simulink model "all_together_simu_v1"  (R2020b)
settings: Solver=FixedStepDiscrete  StartTime=0.0  StopTime=simTime  RelTol=1e-3
InitFcn:
  | generate_locals_for_simulink
values from neighbouring files (symbols this model uses):
  Hh = abs(V(:,1)'*sqrt(S(1,1)))    [setup_old.m]
  Hv = abs(U(:,1)*sqrt(S(1,1)))    [setup_old.m]
undefined symbols (not defined in the file or in its folder): gray, magnitude, Rec, SDTV
libraries: hdlsllib x52, simulink x15, visionhdlio x11, visionsinks x7, visionhdlutilities x4, visionconversions x1, visionsources x1
(part 1 of 2)
settings Model: DataTypeOverride=Off  SimulationMode=accelerator  Creator=The MathWorks, Inc.  LastModifiedBy=Ethan
settings SolverCC: AutoInsertRateTranBlk=on
settings DataIOCC: LimitDataPoints=on  SaveOutput=off  SignalLogging=off  SaveTime=off  ReturnWorkspaceOutputs=off
settings OptimizationCC: BlockReduction=off  ConditionallyExecuteInputs=off  DefaultParameterBehavior=Inlined  LifeSpan=inf
settings DebuggingCC: AlgebraicLoopMsg=error  SingleTaskRateTransMsg=error  ParameterPrecisionLossMsg=none  AllowSymbolicDim=off  StrictBusMsg=ErrorOnBusTreatedAsVector  SFUnexpectedBacktrackingDiag=warning  SFNoUnconditionalDefaultTransitionDiag=warning  SFExecutionAtInitializationDiag=none  ArithmeticOperatorsInVariantConditions=warning
settings HardwareCC: ProdBitPerPointer=32  ProdBitPerSizeT=32  ProdBitPerPtrDiffT=32  ProdLargestAtomicFloat=None  ProdIntDivRoundTo=Undefined  ProdEndianess=Unspecified  ProdWordSize=32  ProdHWDeviceType=ASIC/FPGA->ASIC/FPGA  ProdEqTarget=off
settings SFSimCC: SimUseLocalCustomCode=off  CustomCodeUndefinedFunction=UseInterfaceOnly
settings RTWCC: RTWUseLocalCustomCode=off
settings CodeAppCC: StateflowObjectComments=on
settings GRTTargetCC: TargetLangStandard=C89/C90 (ANSI)
settings ConfigComp: CovMetricSettings=dw  CovSaveCumulativeToWorkspaceVar=on  CovSaveSingleToWorkspaceVar=on  CovExternalEMLEnable=off  CovSFcnEnable=off

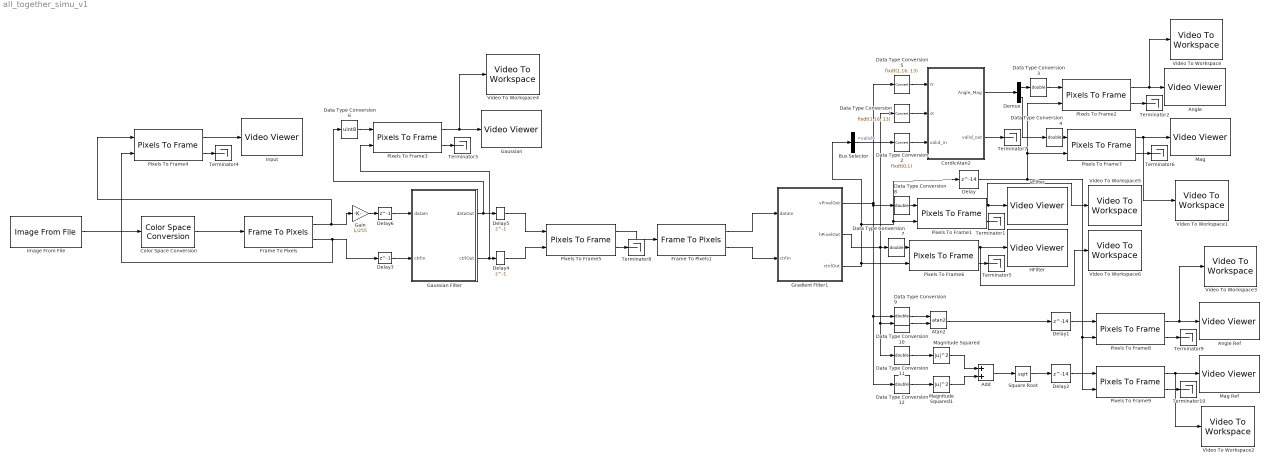
== system all_together_simu_v1 ==
  Add : Sum
  Angle : VideoViewer  colormapValue=gray(256)  FigPos=[1922 517 909 409]
  Angle Ref : VideoViewer  FigPos=[2808 517 958 409]
  Atan2 : Trigonometry  Operator=atan2  ApproximationMethod=CORDIC  NumberOfIterations=12
  Bus Selector : BusSelector  OutputSignals=valid
  Color Space Conversion : visionconversions/Color Space  Conversion  conversion=Obsolete  conversionActive=R'G'B' to intensity  wp_str=D65  rec=Rec. 601 (SDTV)  sys=1125/60/2:1  imagePorts=One multidimensional signal
  CordicAtan2 : Subsystem
  Data Type Conversion1 : DataTypeConversion  OutMin=0  OutMax=1  OutDataTypeStr=fixdt(1,16, 13)
  Data Type Conversion{7..12} (6 alike) : DataTypeConversion  OutMin=0  OutMax=1  OutDataTypeStr=double
  Data Type Conversion2 : DataTypeConversion  OutMin=0  OutMax=1  OutDataTypeStr=fixdt(0,1)
  Data Type Conversion3 : DataTypeConversion  OutDataTypeStr=double
  Data Type Conversion4 : DataTypeConversion  OutDataTypeStr=double
  Data Type Conversion5 : DataTypeConversion  OutMin=0  OutMax=1  OutDataTypeStr=fixdt(1,16, 13)
  Data Type Conversion6 : DataTypeConversion  OutMin=0  OutMax=1  OutDataTypeStr=uint8
  Delay : Delay  DelayLength=14
  Delay1 : Delay  DelayLength=14
  Delay2 : Delay  DelayLength=14
  Delay{3..6} (4 alike) : Delay  DelayLength=1
  Demux : Demux  Outputs=2
  Frame To Pixels : visionhdlio/Frame To Pixels  NumComponents=1  NumPixels=1  VideoFormat=480p  ActivePixelsPerLine=32  ActiveVideoLines=18  TotalPixelsPerLine=42  TotalVideoLines=28  StartingActiveLine=6  FrontPorch=5  SampleTime=0
      settings: SourceProductName=Vision HDL Toolbox
  Frame To Pixels1 : visionhdlio/Frame To Pixels  NumComponents=1  NumPixels=1  VideoFormat=480p  ActivePixelsPerLine=32  ActiveVideoLines=18  TotalPixelsPerLine=42  TotalVideoLines=28  StartingActiveLine=6  FrontPorch=5  SampleTime=0
      settings: SourceProductName=Vision HDL Toolbox
  Gain : Gain  Gain=1/255  OutDataTypeStr=fixdt(1,16, 14)
  Gaussian : VideoViewer  FigPos=[2900 799 813 623.666666666667]
  Gaussian Filter : Subsystem
  Gradient Filter1 : Subsystem
  HFilter : VideoViewer  FigPos=[2895 936 813 624]
  Image From File : visionsources/Image From File  Tag=vipblks_nd  FileName=start.png  Ts=1  imagePorts=One multidimensional signal  OutPortLabels=R|G|B  ImageDataType=uint8  sdImageDataType=uint(8)  Signed=on  WordLength=16  FractionLengthMode=User-defined  FractionLength=15
  Input : VideoViewer  FigPos=[170 848 670 624]
  Mag : VideoViewer  FigPos=[1914 1017 954 411]
  Mag Ref : VideoViewer  FigPos=[2855 1015 954 411]
  Magnitude Squared : Math  Operator=magnitude^2  SaturateOnIntegerOverflow=on
  Magnitude Squared1 : Math  Operator=magnitude^2  SaturateOnIntegerOverflow=on
  Pixels To Frame{1..9} (9 alike) : visionhdlio/Pixels To Frame  NumComponents=1  NumPixels=1  VideoFormat=480p  ActivePixelsPerLine=32  ActiveVideoLines=18  TotalPixelsPerLine=42  TotalVideoLines=28
      settings: SourceProductBaseCode=VT
  Square Root : Sqrt  SaturateOnIntegerOverflow=on
  Terminator{1..10} (10 alike) : Terminator
  VFilter : VideoViewer  FigPos=[928 938 813 624]
  Video To Workspace : visionsinks/Video To Workspace  VariableName=angle  NumInputs=1  DataLimit=10  DecimationFactor=1  LogFi=off  InPortLabels=R|G|B
      settings: SourceProductBaseCode=VP
  Video To Workspace1 : visionsinks/Video To Workspace  VariableName=mag  NumInputs=1  DataLimit=10  DecimationFactor=1  LogFi=off  InPortLabels=R|G|B
      settings: SourceProductBaseCode=VP
  Video To Workspace2 : visionsinks/Video To Workspace  VariableName=mag_ref  NumInputs=1  DataLimit=10  DecimationFactor=1  LogFi=off  InPortLabels=R|G|B
      settings: SourceProductBaseCode=VP
  Video To Workspace3 : visionsinks/Video To Workspace  VariableName=angle_ref  NumInputs=1  DataLimit=10  DecimationFactor=1  LogFi=off  InPortLabels=R|G|B
      settings: SourceProductBaseCode=VP
  Video To Workspace4 : visionsinks/Video To Workspace  VariableName=gaussian  NumInputs=1  DataLimit=10  DecimationFactor=1  LogFi=off  InPortLabels=R|G|B
      settings: SourceProductBaseCode=VP
  Video To Workspace5 : visionsinks/Video To Workspace  VariableName=iy  NumInputs=1  DataLimit=10  DecimationFactor=1  LogFi=off  InPortLabels=R|G|B
      settings: SourceProductBaseCode=VP
  Video To Workspace6 : visionsinks/Video To Workspace  VariableName=ix  NumInputs=1  DataLimit=10  DecimationFactor=1  LogFi=off  InPortLabels=R|G|B
      settings: SourceProductBaseCode=VP
  wires:
  Delay6/1 -> Gaussian Filter/1(dataIn)
  Delay3/1 -> Gaussian Filter/2(ctrlIn)
  Gaussian Filter/2(ctrlOut) -> Pixels To Frame3/2, Delay4/1
  Frame To Pixels/2 -> Pixels To Frame4/2, Delay3/1
  Pixels To Frame3/1 -> Video To Workspace4/1, Gaussian/1
  Pixels To Frame3/2 -> Terminator3/1
  Gaussian Filter/1(dataOut) -> Data Type Conversion6/1, Delay5/1
  Pixels To Frame4/2 -> Terminator4/1
  Pixels To Frame4/1 -> Input/1
  Frame To Pixels/1 -> Pixels To Frame4/1, Gain/1
  Pixels To Frame1/2 -> Terminator1/1
  Pixels To Frame1/1 -> Video To Workspace5/1, VFilter/1
  Gradient Filter1/3(ctrilOut) -> Pixels To Frame6/2, Bus Selector/1, Delay/1, Pixels To Frame1/2
  Delay5/1 -> Pixels To Frame5/1
  Delay4/1 -> Pixels To Frame5/2
  Pixels To Frame5/1 -> Frame To Pixels1/1
  Frame To Pixels1/1 -> Gradient Filter1/1(dataIn)
  Frame To Pixels1/2 -> Gradient Filter1/2(ctrlIn)
  Pixels To Frame6/1 -> HFilter/1, Video To Workspace6/1
  Pixels To Frame6/2 -> Terminator5/1
  Bus Selector/1 -> Data Type Conversion2/1  "<valid>"
  Pixels To Frame2/2 -> Terminator2/1
  Pixels To Frame2/1 -> Video To Workspace/1, Angle/1
  CordicAtan2/1(Angle_Mag) -> Demux/1
  Demux/1 -> Data Type Conversion3/1
  Pixels To Frame7/2 -> Terminator6/1
  Pixels To Frame7/1 -> Video To Workspace1/1, Mag/1
  Demux/2 -> Data Type Conversion4/1
  Delay/1 -> Pixels To Frame9/2, Pixels To Frame8/2, Pixels To Frame2/2, Pixels To Frame7/2
  CordicAtan2/2(valid_out) -> Terminator7/1
  Pixels To Frame5/2 -> Terminator8/1
  Data Type Conversion3/1 -> Pixels To Frame2/1
  Data Type Conversion4/1 -> Pixels To Frame7/1
  Gain/1 -> Delay6/1
  Data Type Conversion2/1 -> CordicAtan2/3(valid_in)
  Atan2/1 -> Delay1/1
  Magnitude Squared/1 -> Add/1
  Magnitude Squared1/1 -> Add/2
  Add/1 -> Square Root/1
  Square Root/1 -> Delay2/1
  Delay2/1 -> Pixels To Frame9/1
  Delay1/1 -> Pixels To Frame8/1
  Pixels To Frame9/1 -> Video To Workspace2/1, Mag Ref/1
  Pixels To Frame8/1 -> Video To Workspace3/1, Angle Ref/1
  Pixels To Frame8/2 -> Terminator9/1
  Pixels To Frame9/2 -> Terminator10/1
  Image From File/1 -> Color Space Conversion/1
  Color Space Conversion/1 -> Frame To Pixels/1
  Gradient Filter1/2(hPixelOut) -> Data Type Conversion1/1, Data Type Conversion7/1, Data Type Conversion11/1, Data Type Conversion10/1
  Gradient Filter1/1(vPixelOut) -> Data Type Conversion5/1, Data Type Conversion8/1, Data Type Conversion9/1, Data Type Conversion12/1
  Data Type Conversion6/1 -> Pixels To Frame3/1
  Data Type Conversion7/1 -> Pixels To Frame6/1
  Data Type Conversion8/1 -> Pixels To Frame1/1
  Data Type Conversion9/1 -> Atan2/1
  Data Type Conversion10/1 -> Atan2/2
  Data Type Conversion11/1 -> Magnitude Squared/1
  Data Type Conversion12/1 -> Magnitude Squared1/1
  Data Type Conversion1/1 -> CordicAtan2/2(iX)
  Data Type Conversion5/1 -> CordicAtan2/1(iY)

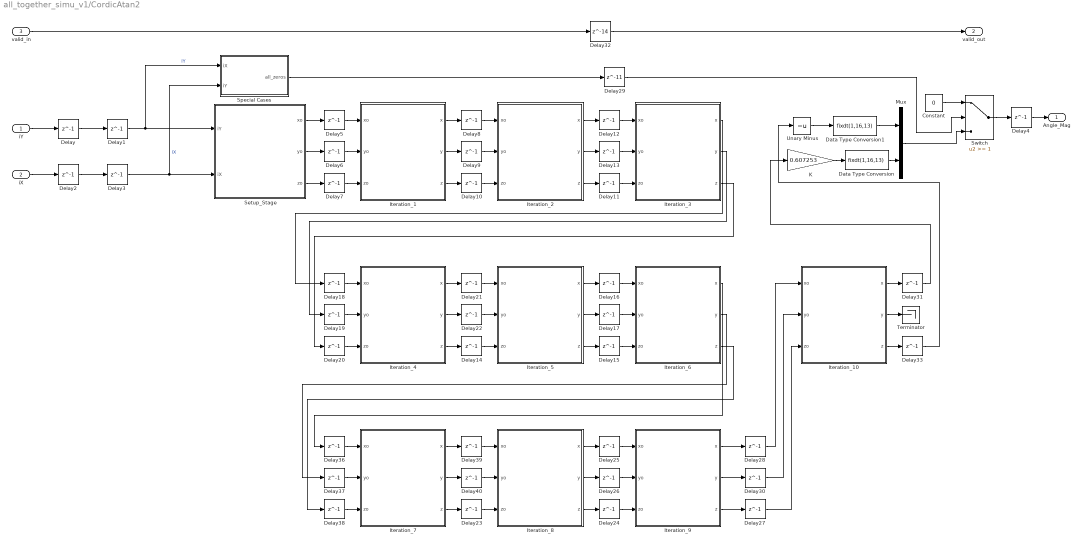
== system all_together_simu_v1/CordicAtan2 ==
  iY : Inport
  iX : Inport  Port=2
  valid_in : Inport  Port=3  OutMin=[0]  OutMax=[1]  OutDataTypeStr=fixdt(0,1)
  Constant : Constant  Value=0  OutDataTypeStr=fixdt(1,16,14)  SampleTime=-1
  Data Type Conversion : DataTypeConversion  OutDataTypeStr=fixdt(1,16,13)
  Data Type Conversion1 : DataTypeConversion  OutDataTypeStr=fixdt(1,16,13)
  Delay{,1..28,30..31,33,36..40} (37 alike) : Delay  DelayLength=1
  Delay29 : Delay  DelayLength=11
  Delay32 : Delay  DelayLength=14
  Iteration_1 : Subsystem
  Iteration_10 : Subsystem
  Iteration_2 : Subsystem
  Iteration_3 : Subsystem
  Iteration_4 : Subsystem
  Iteration_5 : Subsystem
  Iteration_6 : Subsystem
  Iteration_7 : Subsystem
  Iteration_8 : Subsystem
  Iteration_9 : Subsystem
  K : Gain  Gain=0.607253  OutDataTypeStr=Inherit: Inherit via back propagation
  Mux : Mux  Inputs=2
  Setup_Stage : Subsystem
  Special Cases : Subsystem
  Switch : Switch  Threshold=1
  Terminator : Terminator
  Unary Minus : UnaryMinus
  Angle_Mag : Outport
  valid_out : Outport  Port=2  OutMin=[0]  OutMax=[1]  OutDataTypeStr=fixdt(0,1)
  wires:
  iY/1 -> Delay/1
  Delay/1 -> Delay1/1
  Delay2/1 -> Delay3/1
  iX/1 -> Delay2/1
  Constant/1 -> Switch/1
  Delay4/1 -> Angle_Mag/1
  Switch/1 -> Delay4/1
  Delay1/1 -> Setup_Stage/1(iY), Special Cases/1(iX)  "iY"
  Delay3/1 -> Special Cases/2(iY), Setup_Stage/2(iX)  "iX"
  Special Cases/1(all_zeros) -> Delay29/1
  Setup_Stage/1(xo) -> Delay5/1
  Setup_Stage/2(yo) -> Delay6/1
  Setup_Stage/3(zo) -> Delay7/1
  Delay7/1 -> Iteration_1/3(zo)
  Delay6/1 -> Iteration_1/2(yo)
  Delay5/1 -> Iteration_1/1(xo)
  Iteration_1/3(z) -> Delay10/1
  Iteration_1/1(x) -> Delay8/1
  Iteration_1/2(y) -> Delay9/1
  Delay9/1 -> Iteration_2/2(yo)
  Delay10/1 -> Iteration_2/3(zo)
  Delay8/1 -> Iteration_2/1(xo)
  Delay11/1 -> Iteration_3/3(zo)
  Delay12/1 -> Iteration_3/1(xo)
  Delay13/1 -> Iteration_3/2(yo)
  Iteration_2/2(y) -> Delay13/1
  Iteration_2/1(x) -> Delay12/1
  Iteration_2/3(z) -> Delay11/1
  Iteration_5/1(x) -> Delay16/1
  Iteration_5/2(y) -> Delay17/1
  Delay16/1 -> Iteration_6/1(xo)
  Delay17/1 -> Iteration_6/2(yo)
  Delay15/1 -> Iteration_6/3(zo)
  Iteration_5/3(z) -> Delay15/1
  Iteration_4/3(z) -> Delay14/1
  Delay14/1 -> Iteration_5/3(zo)
  Iteration_4/2(y) -> Delay22/1
  Delay21/1 -> Iteration_5/1(xo)
  Delay18/1 -> Iteration_4/1(xo)
  Delay20/1 -> Iteration_4/3(zo)
  Iteration_4/1(x) -> Delay21/1
  Delay22/1 -> Iteration_5/2(yo)
  Delay19/1 -> Iteration_4/2(yo)
  Iteration_8/1(x) -> Delay25/1
  Iteration_8/2(y) -> Delay26/1
  Delay25/1 -> Iteration_9/1(xo)
  Delay26/1 -> Iteration_9/2(yo)
  Delay24/1 -> Iteration_9/3(zo)
  Iteration_8/3(z) -> Delay24/1
  Iteration_7/3(z) -> Delay23/1
  Delay23/1 -> Iteration_8/3(zo)
  Iteration_7/2(y) -> Delay40/1
  Delay39/1 -> Iteration_8/1(xo)
  Delay36/1 -> Iteration_7/1(xo)
  Delay38/1 -> Iteration_7/3(zo)
  Iteration_7/1(x) -> Delay39/1
  Delay40/1 -> Iteration_8/2(yo)
  Delay37/1 -> Iteration_7/2(yo)
  Iteration_3/3(z) -> Delay20/1
  Iteration_3/2(y) -> Delay19/1
  Iteration_3/1(x) -> Delay18/1
  Iteration_6/3(z) -> Delay38/1
  Iteration_6/2(y) -> Delay37/1
  Iteration_6/1(x) -> Delay36/1
  Iteration_9/2(y) -> Delay30/1
  Iteration_9/1(x) -> Delay28/1
  Iteration_9/3(z) -> Delay27/1
  Mux/1 -> Switch/3
  Delay29/1 -> Switch/2
  Delay28/1 -> Iteration_10/1(xo)
  Delay30/1 -> Iteration_10/2(yo)
  Delay27/1 -> Iteration_10/3(zo)
  Iteration_10/1(x) -> Delay31/1
  Delay31/1 -> K/1
  Iteration_10/2(y) -> Terminator/1
  Iteration_10/3(z) -> Delay33/1
  Delay33/1 -> Unary Minus/1
  Unary Minus/1 -> Data Type Conversion1/1
  valid_in/1 -> Delay32/1
  Delay32/1 -> valid_out/1
  Data Type Conversion/1 -> Mux/2
  K/1 -> Data Type Conversion/1
  Data Type Conversion1/1 -> Mux/1

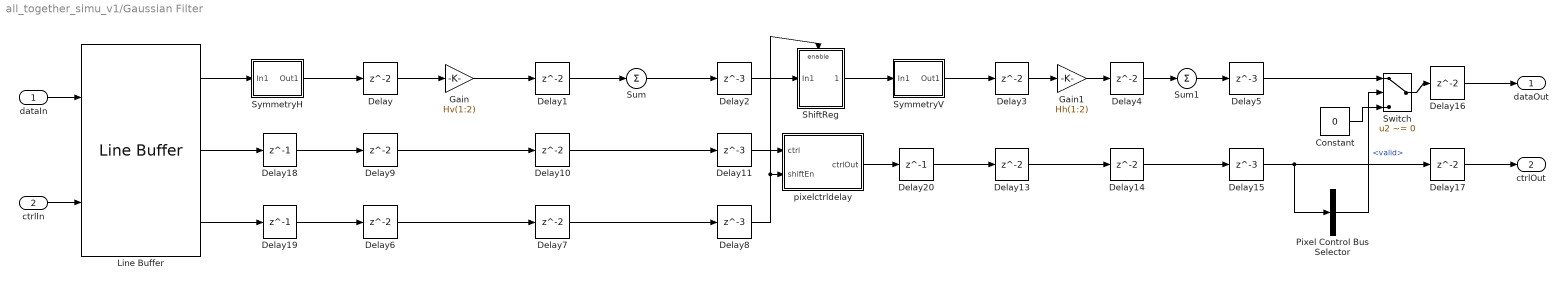
== system all_together_simu_v1/Gaussian Filter ==
  dataIn : Inport
  ctrlIn : Inport  Port=2
  Constant : Constant  Value=0  OutDataTypeStr=Inherit: Inherit via back propagation  SampleTime=-1
  Delay{,1,3..4,6..7,9..10,13..14,16..17} (12 alike) : Delay
  Delay{2,5,8,11,15} (5 alike) : Delay  DelayLength=3
  Delay18 : Delay  DelayLength=1
  Delay19 : Delay  DelayLength=1
  Delay20 : Delay  DelayLength=1
  Gain : Gain  Gain=Hv(1:2)  ParamDataTypeStr=good_fixdt
  Gain1 : Gain  Gain=Hh(1:2)  ParamDataTypeStr=good_fixdt
  Line Buffer : visionhdlutilities/Line Buffer  NeighborhoodSize=[3 3]  PaddingMethod=None  PaddingValue=0  LineBufferSize=2048  SimulateUsing=Code generation
      settings: SourceProductName=Vision HDL Toolbox
  Pixel Control Bus Selector : BusSelector  OutputSignals=valid
  ShiftReg : Subsystem
  Sum : Sum  Inputs=1  OutDataTypeStr=Inherit: Same as accumulator
  Sum1 : Sum  Inputs=1  OutDataTypeStr=Inherit: Same as accumulator
  Switch : Switch  Criteria=u2 ~= 0
  SymmetryH : Subsystem
  SymmetryV : Subsystem
  pixelctrldelay : Subsystem
  dataOut : Outport  VectorParamsAs1DForOutWhenUnconnected=off
  ctrlOut : Outport  Port=2  VectorParamsAs1DForOutWhenUnconnected=off
  wires:
  Gain/1 -> Delay1/1
  Delay8/1 -> pixelctrldelay/2(shiftEn), ShiftReg/Enable
  Delay3/1 -> Gain1/1
  Sum/1 -> Delay2/1
  Gain1/1 -> Delay4/1
  Sum1/1 -> Delay5/1
  Delay9/1 -> Delay10/1
  dataIn/1 -> Line Buffer/1
  Delay10/1 -> Delay11/1
  Delay4/1 -> Sum1/1
  Delay6/1 -> Delay7/1
  Delay1/1 -> Sum/1
  Delay17/1 -> ctrlOut/1
  Constant/1 -> Switch/3
  Delay14/1 -> Delay15/1
  Delay13/1 -> Delay14/1
  Delay2/1 -> ShiftReg/1(In1)
  Delay7/1 -> Delay8/1
  Switch/1 -> Delay16/1
  Delay15/1 -> Delay17/1, Pixel Control Bus Selector/1
  Pixel Control Bus Selector/1 -> Switch/2  "<valid>"
  Delay/1 -> Gain/1
  ctrlIn/1 -> Line Buffer/2
  Delay16/1 -> dataOut/1
  Line Buffer/3 -> Delay19/1
  Line Buffer/2 -> Delay18/1
  ShiftReg/1(Out1) -> SymmetryV/1(In1)
  Line Buffer/1 -> SymmetryH/1(In1)
  SymmetryH/1(Out1) -> Delay/1
  Delay18/1 -> Delay9/1
  Delay19/1 -> Delay6/1
  SymmetryV/1(Out1) -> Delay3/1
  Delay20/1 -> Delay13/1
  Delay11/1 -> pixelctrldelay/1(ctrl)
  pixelctrldelay/1(ctrlOut) -> Delay20/1
  Delay5/1 -> Switch/1

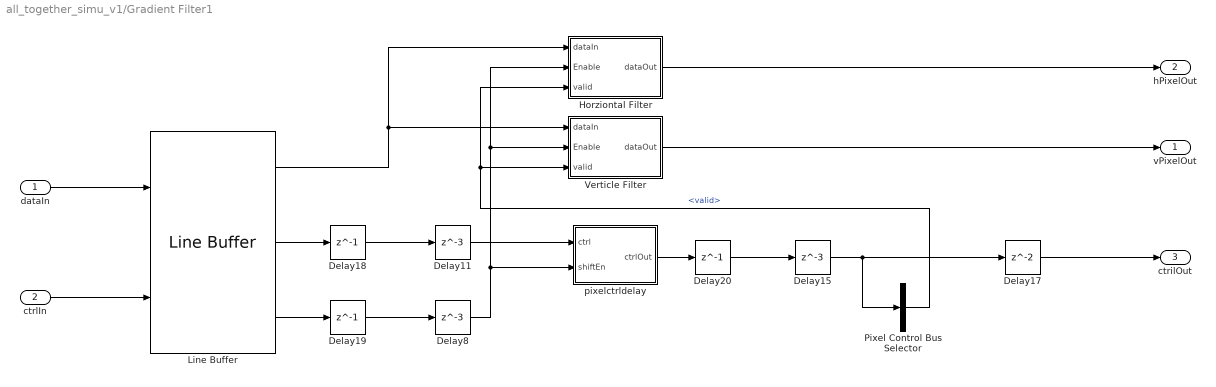
== system all_together_simu_v1/Gradient Filter1 ==
  dataIn : Inport
  ctrlIn : Inport  Port=2
  Delay11 : Delay  DelayLength=3
  Delay15 : Delay  DelayLength=3
  Delay17 : Delay
  Delay18 : Delay  DelayLength=1
  Delay19 : Delay  DelayLength=1
  Delay20 : Delay  DelayLength=1
  Delay8 : Delay  DelayLength=3
  Horziontal Filter : Subsystem
  Line Buffer : visionhdlutilities/Line Buffer  NeighborhoodSize=[3 3]  PaddingMethod=None  PaddingValue=0  LineBufferSize=2048  SimulateUsing=Code generation
      settings: SourceProductName=Vision HDL Toolbox
  Pixel Control Bus Selector : BusSelector  OutputSignals=valid
  Verticle Filter : Subsystem
  pixelctrldelay : Subsystem
  vPixelOut : Outport  VectorParamsAs1DForOutWhenUnconnected=off
  hPixelOut : Outport  Port=2  VectorParamsAs1DForOutWhenUnconnected=off
  ctrilOut : Outport  Port=3  VectorParamsAs1DForOutWhenUnconnected=off
  wires:
  ctrlIn/1 -> Line Buffer/2
  dataIn/1 -> Line Buffer/1
  Line Buffer/1 -> Horziontal Filter/1(dataIn), Verticle Filter/1(dataIn)
  Delay20/1 -> Delay15/1
  Delay19/1 -> Delay8/1
  Delay11/1 -> pixelctrldelay/1(ctrl)
  pixelctrldelay/1(ctrlOut) -> Delay20/1
  Delay15/1 -> Delay17/1, Pixel Control Bus Selector/1
  Delay18/1 -> Delay11/1
  Delay8/1 -> Horziontal Filter/2(Enable), Verticle Filter/2(Enable), pixelctrldelay/2(shiftEn)
  Line Buffer/2 -> Delay18/1
  Line Buffer/3 -> Delay19/1
  Pixel Control Bus Selector/1 -> Horziontal Filter/3(valid), Verticle Filter/3(valid)  "<valid>"
  Verticle Filter/1(dataOut) -> vPixelOut/1
  Horziontal Filter/1(dataOut) -> hPixelOut/1
  Delay17/1 -> ctrilOut/1

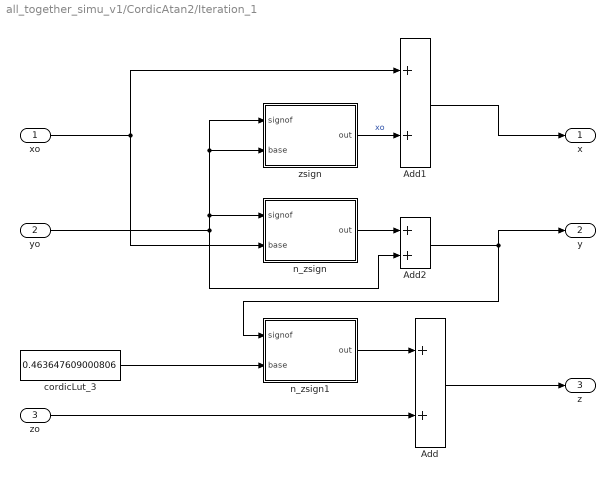
== system all_together_simu_v1/CordicAtan2/Iteration_1 ==
  xo : Inport
  yo : Inport  Port=2
  zo : Inport  Port=3
  Add : Sum
  Add1 : Sum
  Add2 : Sum
  cordicLut_3 : Constant  Value=0.463647609000806  OutDataTypeStr=fixdt(1,16,16)  SampleTime=-1
  n_zsign : Subsystem
  n_zsign1 : Subsystem
  zsign : Subsystem
  x : Outport
  y : Outport  Port=2
  z : Outport  Port=3
  wires:
  Add/1 -> z/1
  cordicLut_3/1 -> n_zsign1/2(base)
  zo/1 -> Add/2
  n_zsign1/1(out) -> Add/1
  yo/1 -> zsign/2(base), zsign/1(signof), n_zsign/1(signof), Add2/2
  zsign/1(out) -> Add1/2  "xo"
  xo/1 -> n_zsign/2(base), Add1/1
  Add1/1 -> x/1
  n_zsign/1(out) -> Add2/1
  Add2/1 -> n_zsign1/1(signof), y/1

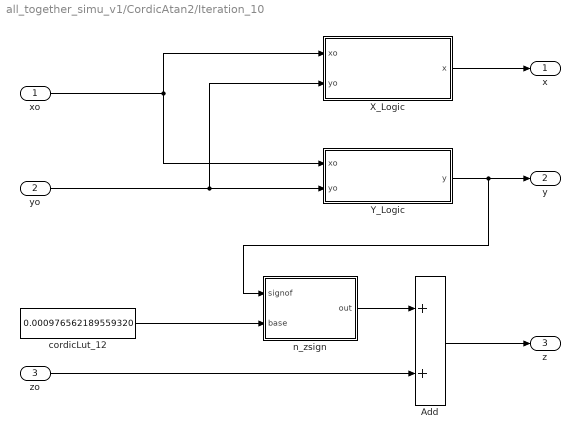
== system all_together_simu_v1/CordicAtan2/Iteration_10 ==
  xo : Inport
  yo : Inport  Port=2
  zo : Inport  Port=3
  Add : Sum
  X_Logic : Subsystem
  Y_Logic : Subsystem
  cordicLut_12 : Constant  Value=0.000976562189559320  OutDataTypeStr=fixdt(1,16,24)  SampleTime=-1
  n_zsign : Subsystem
  x : Outport
  y : Outport  Port=2
  z : Outport  Port=3
  wires:
  Add/1 -> z/1
  cordicLut_12/1 -> n_zsign/2(base)
  zo/1 -> Add/2
  n_zsign/1(out) -> Add/1
  yo/1 -> Y_Logic/2(yo), X_Logic/2(yo)
  xo/1 -> Y_Logic/1(xo), X_Logic/1(xo)
  X_Logic/1(x) -> x/1
  Y_Logic/1(y) -> n_zsign/1(signof), y/1

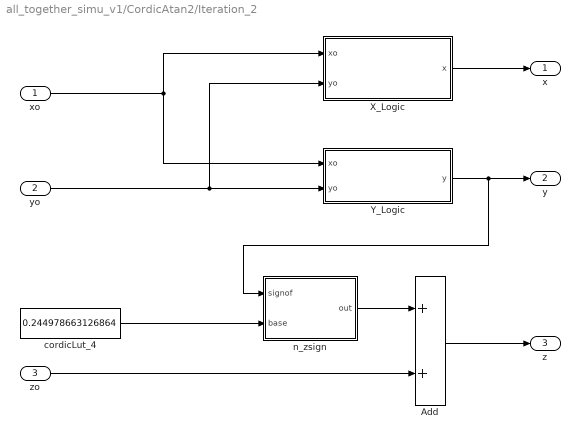
== system all_together_simu_v1/CordicAtan2/Iteration_2 ==
  xo : Inport
  yo : Inport  Port=2
  zo : Inport  Port=3
  Add : Sum
  X_Logic : Subsystem
  Y_Logic : Subsystem
  cordicLut_4 : Constant  Value=0.244978663126864  OutDataTypeStr=fixdt(1,16, 17)  SampleTime=-1
  n_zsign : Subsystem
  x : Outport
  y : Outport  Port=2
  z : Outport  Port=3
  wires:
  Add/1 -> z/1
  cordicLut_4/1 -> n_zsign/2(base)
  zo/1 -> Add/2
  n_zsign/1(out) -> Add/1
  yo/1 -> Y_Logic/2(yo), X_Logic/2(yo)
  xo/1 -> Y_Logic/1(xo), X_Logic/1(xo)
  X_Logic/1(x) -> x/1
  Y_Logic/1(y) -> n_zsign/1(signof), y/1

== system all_together_simu_v1/CordicAtan2/Iteration_3 ==
  xo : Inport
  yo : Inport  Port=2
  zo : Inport  Port=3
  Add : Sum
  X_Logic : Subsystem
  Y_Logic : Subsystem
  cordicLut_5 : Constant  Value=0.124354994546761  OutDataTypeStr=fixdt(1,16,17)  SampleTime=-1
  n_zsign : Subsystem
  x : Outport
  y : Outport  Port=2
  z : Outport  Port=3
  wires:
  Add/1 -> z/1
  cordicLut_5/1 -> n_zsign/2(base)
  zo/1 -> Add/2
  n_zsign/1(out) -> Add/1
  yo/1 -> Y_Logic/2(yo), X_Logic/2(yo)
  xo/1 -> Y_Logic/1(xo), X_Logic/1(xo)
  X_Logic/1(x) -> x/1
  Y_Logic/1(y) -> n_zsign/1(signof), y/1

== system all_together_simu_v1/CordicAtan2/Iteration_4 ==
  xo : Inport
  yo : Inport  Port=2
  zo : Inport  Port=3
  Add : Sum
  X_Logic : Subsystem
  Y_Logic : Subsystem
  cordicLut_6 : Constant  Value=0.0624188099959574  OutDataTypeStr=fixdt(1,16,18)  SampleTime=-1
  n_zsign : Subsystem
  x : Outport
  y : Outport  Port=2
  z : Outport  Port=3
  wires:
  Add/1 -> z/1
  cordicLut_6/1 -> n_zsign/2(base)
  zo/1 -> Add/2
  n_zsign/1(out) -> Add/1
  yo/1 -> Y_Logic/2(yo), X_Logic/2(yo)
  xo/1 -> Y_Logic/1(xo), X_Logic/1(xo)
  X_Logic/1(x) -> x/1
  Y_Logic/1(y) -> n_zsign/1(signof), y/1

== system all_together_simu_v1/CordicAtan2/Iteration_5 ==
  xo : Inport
  yo : Inport  Port=2
  zo : Inport  Port=3
  Add : Sum
  X_Logic : Subsystem
  Y_Logic : Subsystem
  cordicLut_7 : Constant  Value=0.0312398334302683  OutDataTypeStr=fixdt(1,16,19)  SampleTime=-1
  n_zsign : Subsystem
  x : Outport
  y : Outport  Port=2
  z : Outport  Port=3
  wires:
  Add/1 -> z/1
  cordicLut_7/1 -> n_zsign/2(base)
  zo/1 -> Add/2
  n_zsign/1(out) -> Add/1
  yo/1 -> Y_Logic/2(yo), X_Logic/2(yo)
  xo/1 -> Y_Logic/1(xo), X_Logic/1(xo)
  X_Logic/1(x) -> x/1
  Y_Logic/1(y) -> n_zsign/1(signof), y/1

== system all_together_simu_v1/CordicAtan2/Iteration_6 ==
  xo : Inport
  yo : Inport  Port=2
  zo : Inport  Port=3
  Add : Sum
  X_Logic : Subsystem
  Y_Logic : Subsystem
  cordicLut_8 : Constant  Value=0.0156237286204768  OutDataTypeStr=fixdt(1,16,20)  SampleTime=-1
  n_zsign : Subsystem
  x : Outport
  y : Outport  Port=2
  z : Outport  Port=3
  wires:
  Add/1 -> z/1
  cordicLut_8/1 -> n_zsign/2(base)
  zo/1 -> Add/2
  n_zsign/1(out) -> Add/1
  yo/1 -> Y_Logic/2(yo), X_Logic/2(yo)
  xo/1 -> Y_Logic/1(xo), X_Logic/1(xo)
  X_Logic/1(x) -> x/1
  Y_Logic/1(y) -> n_zsign/1(signof), y/1

== system all_together_simu_v1/CordicAtan2/Iteration_7 ==
  xo : Inport
  yo : Inport  Port=2
  zo : Inport  Port=3
  Add : Sum
  X_Logic : Subsystem
  Y_Logic : Subsystem
  cordicLut_9 : Constant  Value=0.00781234106010111  OutDataTypeStr=fixdt(1,16,21)  SampleTime=-1
  n_zsign : Subsystem
  x : Outport
  y : Outport  Port=2
  z : Outport  Port=3
  wires:
  Add/1 -> z/1
  cordicLut_9/1 -> n_zsign/2(base)
  zo/1 -> Add/2
  n_zsign/1(out) -> Add/1
  yo/1 -> Y_Logic/2(yo), X_Logic/2(yo)
  xo/1 -> Y_Logic/1(xo), X_Logic/1(xo)
  X_Logic/1(x) -> x/1
  Y_Logic/1(y) -> n_zsign/1(signof), y/1

== system all_together_simu_v1/CordicAtan2/Iteration_8 ==
  xo : Inport
  yo : Inport  Port=2
  zo : Inport  Port=3
  Add : Sum
  X_Logic : Subsystem
  Y_Logic : Subsystem
  cordicLut_10 : Constant  Value=0.00390623013196697  OutDataTypeStr=fixdt(1,16,22)  SampleTime=-1
  n_zsign : Subsystem
  x : Outport
  y : Outport  Port=2
  z : Outport  Port=3
  wires:
  Add/1 -> z/1
  cordicLut_10/1 -> n_zsign/2(base)
  zo/1 -> Add/2
  n_zsign/1(out) -> Add/1
  yo/1 -> Y_Logic/2(yo), X_Logic/2(yo)
  xo/1 -> Y_Logic/1(xo), X_Logic/1(xo)
  X_Logic/1(x) -> x/1
  Y_Logic/1(y) -> n_zsign/1(signof), y/1

== system all_together_simu_v1/CordicAtan2/Iteration_9 ==
  xo : Inport
  yo : Inport  Port=2
  zo : Inport  Port=3
  Add : Sum
  X_Logic : Subsystem
  Y_Logic : Subsystem
  cordicLut_11 : Constant  Value=0.00195312251647882  OutDataTypeStr=fixdt(1,16,23)  SampleTime=-1
  n_zsign : Subsystem
  x : Outport
  y : Outport  Port=2
  z : Outport  Port=3
  wires:
  Add/1 -> z/1
  cordicLut_11/1 -> n_zsign/2(base)
  zo/1 -> Add/2
  n_zsign/1(out) -> Add/1
  yo/1 -> Y_Logic/2(yo), X_Logic/2(yo)
  xo/1 -> Y_Logic/1(xo), X_Logic/1(xo)
  X_Logic/1(x) -> x/1
  Y_Logic/1(y) -> n_zsign/1(signof), y/1

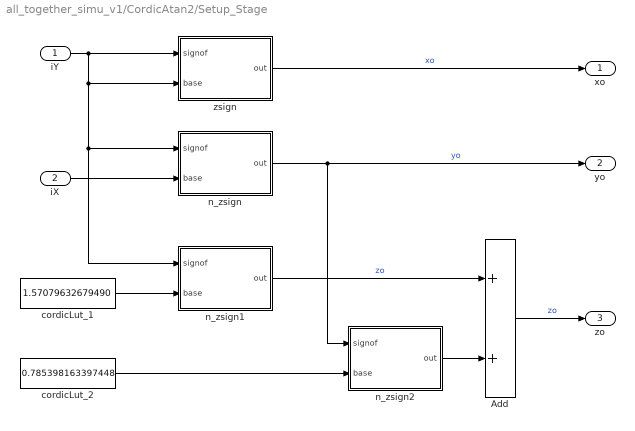
== system all_together_simu_v1/CordicAtan2/Setup_Stage ==
  iY : Inport
  iX : Inport  Port=2
  Add : Sum
  cordicLut_1 : Constant  Value=1.57079632679490  OutDataTypeStr=fixdt(1,16, 14)  SampleTime=-1
  cordicLut_2 : Constant  Value=0.785398163397448  OutDataTypeStr=fixdt(1,16, 15)  SampleTime=-1
  n_zsign : Subsystem
  n_zsign1 : Subsystem
  n_zsign2 : Subsystem
  zsign : Subsystem
  xo : Outport
  yo : Outport  Port=2
  zo : Outport  Port=3
  wires:
  cordicLut_1/1 -> n_zsign1/2(base)
  iY/1 -> zsign/2(base), n_zsign1/1(signof), n_zsign/1(signof), zsign/1(signof)
  n_zsign/1(out) -> n_zsign2/1(signof), yo/1  "yo"
  n_zsign1/1(out) -> Add/1  "zo"
  cordicLut_2/1 -> n_zsign2/2(base)
  iX/1 -> n_zsign/2(base)
  n_zsign2/1(out) -> Add/2
  Add/1 -> zo/1  "zo"
  zsign/1(out) -> xo/1  "xo"

== system all_together_simu_v1/CordicAtan2/Special Cases ==
  iX : Inport
  iY : Inport  Port=2
  Compare To Zero : simulink/Logic and Bit Operations/Compare To Zero  relop===  OutDataTypeStr=boolean
  Compare To Zero1 : simulink/Logic and Bit Operations/Compare To Zero  relop===  OutDataTypeStr=boolean
  Logical Operator : Logic  AllPortsSameDT=off  OutDataTypeStr=boolean
  all_zeros : Outport
  wires:
  Compare To Zero1/1 -> Logical Operator/2
  Logical Operator/1 -> all_zeros/1
  iY/1 -> Compare To Zero1/1
  Compare To Zero/1 -> Logical Operator/1
  iX/1 -> Compare To Zero/1

== system all_together_simu_v1/Gaussian Filter/ShiftReg ==
  In1 : Inport
  Enable : EnablePort
  State Control : StateControl  StateControl=Synchronous
  Tapped Delay : simulink/Discrete/Tapped Delay  vinit=0.0  samptime=-1  NumDelays=3  DelayOrder=Oldest  includeCurrent=off
  Out1 : Outport  VectorParamsAs1DForOutWhenUnconnected=off
  wires:
  In1/1 -> Tapped Delay/1
  Tapped Delay/1 -> Out1/1

== system all_together_simu_v1/Gaussian Filter/SymmetryH ==
  In1 : Inport
  Data Type Duplicate : DataTypeDuplicate
  Data Type Conversion1 : DataTypeConversion
  Delay18 : Delay  DelayLength=1
  Demux : Demux  Outputs=3
  Mux : Mux  Inputs=2
  Sum3 : Sum  Inputs=|++
  Out1 : Outport  VectorParamsAs1DForOutWhenUnconnected=off
  wires:
  Mux/1 -> Delay18/1
  Sum3/1 -> Mux/1, Data Type Duplicate/1
  Data Type Conversion1/1 -> Mux/2, Data Type Duplicate/2
  Delay18/1 -> Out1/1
  In1/1 -> Demux/1
  Demux/1 -> Sum3/1
  Demux/3 -> Sum3/2
  Demux/2 -> Data Type Conversion1/1

== system all_together_simu_v1/Gaussian Filter/SymmetryV ==
  In1 : Inport
  Data Type Duplicate : DataTypeDuplicate
  Data Type Conversion1 : DataTypeConversion
  Delay18 : Delay  DelayLength=1
  Demux : Demux  Outputs=3
  Mux : Mux  Inputs=2
  Sum3 : Sum  Inputs=|++
  Out1 : Outport  VectorParamsAs1DForOutWhenUnconnected=off
  wires:
  In1/1 -> Demux/1
  Delay18/1 -> Out1/1
  Data Type Conversion1/1 -> Mux/2, Data Type Duplicate/2
  Sum3/1 -> Mux/1, Data Type Duplicate/1
  Mux/1 -> Delay18/1
  Demux/3 -> Sum3/2
  Demux/1 -> Sum3/1
  Demux/2 -> Data Type Conversion1/1

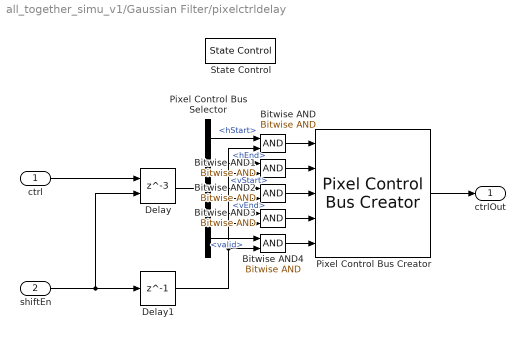
== system all_together_simu_v1/Gaussian Filter/pixelctrldelay ==
  ctrl : Inport
  shiftEn : Inport  Port=2
  Bitwise AND{,1..4} (5 alike) : simulink/Logic and Bit Operations/Bitwise Operator  logicop=AND  UseBitMask=off  NumInputPorts=2  BitMask=bin2dec('11011001')  BitMaskRealWorld=Stored Integer
  Delay : Delay  DelayLength=3  ShowEnablePort=on
      settings: InputPortMap=u0,e6
  Delay1 : Delay  DelayLength=1
  Pixel Control Bus Creator : visionhdlutilities/Pixel Control Bus Creator
      settings: SourceProductName=Vision HDL Toolbox
  Pixel Control Bus Selector : BusSelector  OutputSignals=hStart,hEnd,vStart,vEnd,valid
  State Control : StateControl  StateControl=Synchronous
  ctrlOut : Outport  VectorParamsAs1DForOutWhenUnconnected=off
  wires:
  Bitwise AND4/1 -> Pixel Control Bus Creator/5
  Bitwise AND/1 -> Pixel Control Bus Creator/1
  Pixel Control Bus Selector/3 -> Bitwise AND2/1  "<vStart>"
  Bitwise AND3/1 -> Pixel Control Bus Creator/4
  Pixel Control Bus Selector/5 -> Bitwise AND4/1  "<valid>"
  Delay/1 -> Pixel Control Bus Selector/1
  Pixel Control Bus Selector/1 -> Bitwise AND/1  "<hStart>"
  Pixel Control Bus Selector/2 -> Bitwise AND1/1  "<hEnd>"
  Bitwise AND2/1 -> Pixel Control Bus Creator/3
  Pixel Control Bus Selector/4 -> Bitwise AND3/1  "<vEnd>"
  Bitwise AND1/1 -> Pixel Control Bus Creator/2
  Pixel Control Bus Creator/1 -> ctrlOut/1
  ctrl/1 -> Delay/1
  shiftEn/1 -> Delay1/1, Delay/2
  Delay1/1 -> Bitwise AND3/2, Bitwise AND2/2, Bitwise AND1/2, Bitwise AND/2, Bitwise AND4/2

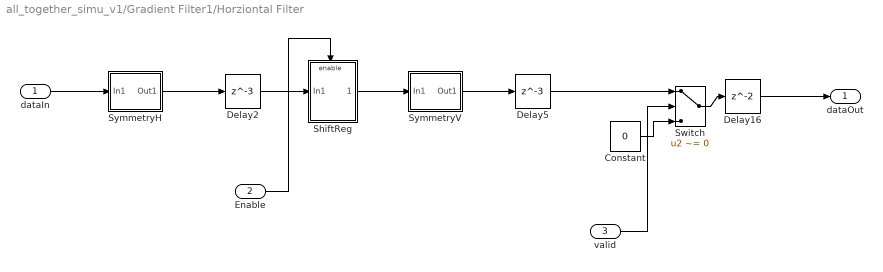
== system all_together_simu_v1/Gradient Filter1/Horziontal Filter ==
  dataIn : Inport
  Enable : Inport  Port=2
  valid : Inport  Port=3
  Constant : Constant  Value=0  OutDataTypeStr=Inherit: Inherit via back propagation  SampleTime=-1
  Delay16 : Delay
  Delay2 : Delay  DelayLength=3
  Delay5 : Delay  DelayLength=3
  ShiftReg : Subsystem
  Switch : Switch  Criteria=u2 ~= 0
  SymmetryH : Subsystem
  SymmetryV : Subsystem
  dataOut : Outport
  wires:
  Switch/1 -> Delay16/1
  ShiftReg/1(Out1) -> SymmetryV/1(In1)
  SymmetryH/1(Out1) -> Delay2/1
  Constant/1 -> Switch/3
  Enable/1 -> ShiftReg/Enable
  SymmetryV/1(Out1) -> Delay5/1
  Delay2/1 -> ShiftReg/1(In1)
  Delay16/1 -> dataOut/1
  Delay5/1 -> Switch/1
  dataIn/1 -> SymmetryH/1(In1)
  valid/1 -> Switch/2

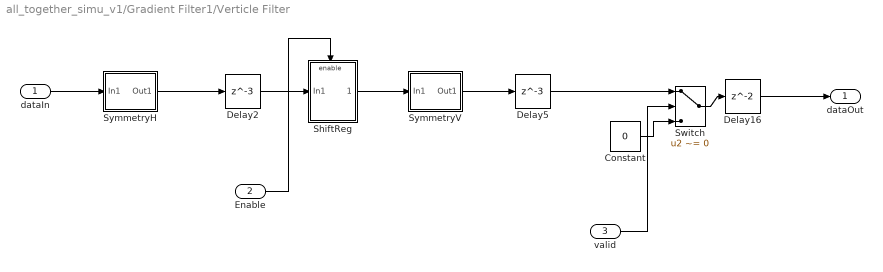
== system all_together_simu_v1/Gradient Filter1/Verticle Filter ==
  dataIn : Inport
  Enable : Inport  Port=2
  valid : Inport  Port=3
  Constant : Constant  Value=0  OutDataTypeStr=Inherit: Inherit via back propagation  SampleTime=-1
  Delay16 : Delay
  Delay2 : Delay  DelayLength=3
  Delay5 : Delay  DelayLength=3
  ShiftReg : Subsystem
  Switch : Switch  Criteria=u2 ~= 0
  SymmetryH : Subsystem
  SymmetryV : Subsystem
  dataOut : Outport
  wires:
  dataIn/1 -> SymmetryH/1(In1)
  Switch/1 -> Delay16/1
  ShiftReg/1(Out1) -> SymmetryV/1(In1)
  Delay2/1 -> ShiftReg/1(In1)
  Delay5/1 -> Switch/1
  SymmetryV/1(Out1) -> Delay5/1
  SymmetryH/1(Out1) -> Delay2/1
  Enable/1 -> ShiftReg/Enable
  Constant/1 -> Switch/3
  valid/1 -> Switch/2
  Delay16/1 -> dataOut/1

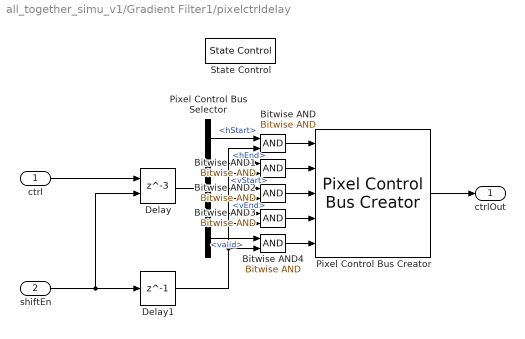
== system all_together_simu_v1/Gradient Filter1/pixelctrldelay ==
  ctrl : Inport
  shiftEn : Inport  Port=2
  Bitwise AND{,1..4} (5 alike) : simulink/Logic and Bit Operations/Bitwise Operator  logicop=AND  UseBitMask=off  NumInputPorts=2  BitMask=bin2dec('11011001')  BitMaskRealWorld=Stored Integer
  Delay : Delay  DelayLength=3  ShowEnablePort=on
      settings: InputPortMap=u0,e6
  Delay1 : Delay  DelayLength=1
  Pixel Control Bus Creator : visionhdlutilities/Pixel Control Bus Creator
      settings: SourceProductName=Vision HDL Toolbox
  Pixel Control Bus Selector : BusSelector  OutputSignals=hStart,hEnd,vStart,vEnd,valid
  State Control : StateControl  StateControl=Synchronous
  ctrlOut : Outport  VectorParamsAs1DForOutWhenUnconnected=off
  wires:
  Bitwise AND4/1 -> Pixel Control Bus Creator/5
  Bitwise AND/1 -> Pixel Control Bus Creator/1
  Pixel Control Bus Selector/3 -> Bitwise AND2/1  "<vStart>"
  Bitwise AND3/1 -> Pixel Control Bus Creator/4
  Pixel Control Bus Selector/5 -> Bitwise AND4/1  "<valid>"
  Delay/1 -> Pixel Control Bus Selector/1
  Pixel Control Bus Selector/1 -> Bitwise AND/1  "<hStart>"
  Pixel Control Bus Selector/2 -> Bitwise AND1/1  "<hEnd>"
  Bitwise AND2/1 -> Pixel Control Bus Creator/3
  Pixel Control Bus Selector/4 -> Bitwise AND3/1  "<vEnd>"
  Bitwise AND1/1 -> Pixel Control Bus Creator/2
  Pixel Control Bus Creator/1 -> ctrlOut/1
  ctrl/1 -> Delay/1
  shiftEn/1 -> Delay1/1, Delay/2
  Delay1/1 -> Bitwise AND3/2, Bitwise AND2/2, Bitwise AND1/2, Bitwise AND/2, Bitwise AND4/2

== system all_together_simu_v1/CordicAtan2/Iteration_1/n_zsign ==
  signof : Inport
  base : Inport  Port=2
  Bit Slice : hdlsllib/Logic and Bit Operations/Bit Slice  lidx=15  ridx=15
      settings: SourceProductBaseCode=SL
  Switch : Switch  Criteria=u2 > Threshold
  Unary Minus : UnaryMinus
  out : Outport
  wires:
  Bit Slice/1 -> Switch/2
  signof/1 -> Bit Slice/1
  base/1 -> Switch/1, Unary Minus/1
  Switch/1 -> out/1
  Unary Minus/1 -> Switch/3

== system all_together_simu_v1/CordicAtan2/Iteration_1/n_zsign1 ==
  signof : Inport
  base : Inport  Port=2
  Bit Slice : hdlsllib/Logic and Bit Operations/Bit Slice  lidx=15  ridx=15
      settings: SourceProductBaseCode=SL
  Switch : Switch  Criteria=u2 > Threshold
  Unary Minus : UnaryMinus
  out : Outport
  wires:
  Bit Slice/1 -> Switch/2
  signof/1 -> Bit Slice/1
  base/1 -> Switch/1, Unary Minus/1
  Switch/1 -> out/1
  Unary Minus/1 -> Switch/3

== system all_together_simu_v1/CordicAtan2/Iteration_1/zsign ==
  signof : Inport
  base : Inport  Port=2
  Bit Slice : hdlsllib/Logic and Bit Operations/Bit Slice  lidx=15  ridx=15
      settings: SourceProductBaseCode=SL
  Switch : Switch  Criteria=u2 > Threshold
  Unary Minus : UnaryMinus
  out : Outport
  wires:
  signof/1 -> Bit Slice/1
  Bit Slice/1 -> Switch/2
  base/1 -> Switch/3, Unary Minus/1
  Switch/1 -> out/1
  Unary Minus/1 -> Switch/1

== system all_together_simu_v1/CordicAtan2/Iteration_10/X_Logic ==
  xo : Inport
  yo : Inport  Port=2
  Add2 : Sum
  Bit Shift : hdlsllib/Logic and Bit Operations/Bit Shift  mode=Shift Right Arithmetic  N=9
  zsign : Subsystem
  x : Outport
  wires:
  yo/1 -> zsign/1(signof), Bit Shift/1
  Bit Shift/1 -> zsign/2(base)
  xo/1 -> Add2/1
  Add2/1 -> x/1
  zsign/1(out) -> Add2/2  "xo"

== system all_together_simu_v1/CordicAtan2/Iteration_10/Y_Logic ==
  xo : Inport
  yo : Inport  Port=2
  Add1 : Sum  OutDataTypeStr=fixdt(1,16,21)
  Bit Shift : hdlsllib/Logic and Bit Operations/Bit Shift  mode=Shift Right Arithmetic  N=9
  n_zsign : Subsystem
  y : Outport
  wires:
  Bit Shift/1 -> n_zsign/2(base)
  n_zsign/1(out) -> Add1/2
  Add1/1 -> y/1
  xo/1 -> Bit Shift/1
  yo/1 -> n_zsign/1(signof), Add1/1

== system all_together_simu_v1/CordicAtan2/Iteration_10/n_zsign ==
  signof : Inport
  base : Inport  Port=2
  Bit Slice : hdlsllib/Logic and Bit Operations/Bit Slice  lidx=15  ridx=15
      settings: SourceProductBaseCode=SL
  Switch : Switch  Criteria=u2 > Threshold
  Unary Minus : UnaryMinus
  out : Outport
  wires:
  Bit Slice/1 -> Switch/2
  signof/1 -> Bit Slice/1
  base/1 -> Switch/1, Unary Minus/1
  Switch/1 -> out/1
  Unary Minus/1 -> Switch/3

== system all_together_simu_v1/CordicAtan2/Iteration_2/X_Logic ==
  xo : Inport
  yo : Inport  Port=2
  Add2 : Sum
  Bit Shift : hdlsllib/Logic and Bit Operations/Bit Shift  mode=Shift Right Arithmetic  N=1
  zsign1 : Subsystem
  x : Outport
  wires:
  yo/1 -> zsign1/1(signof), Bit Shift/1
  Bit Shift/1 -> zsign1/2(base)
  xo/1 -> Add2/1
  Add2/1 -> x/1
  zsign1/1(out) -> Add2/2  "xo"

== system all_together_simu_v1/CordicAtan2/Iteration_2/Y_Logic ==
  xo : Inport
  yo : Inport  Port=2
  Add1 : Sum
  Bit Shift : hdlsllib/Logic and Bit Operations/Bit Shift  mode=Shift Right Arithmetic  N=1
  n_zsign : Subsystem
  y : Outport
  wires:
  Bit Shift/1 -> n_zsign/2(base)
  n_zsign/1(out) -> Add1/2
  Add1/1 -> y/1
  xo/1 -> Bit Shift/1
  yo/1 -> n_zsign/1(signof), Add1/1

== system all_together_simu_v1/CordicAtan2/Iteration_2/n_zsign ==
  signof : Inport
  base : Inport  Port=2
  Bit Slice : hdlsllib/Logic and Bit Operations/Bit Slice  lidx=15  ridx=15
      settings: SourceProductBaseCode=SL
  Switch : Switch  Criteria=u2 > Threshold
  Unary Minus : UnaryMinus
  out : Outport
  wires:
  Bit Slice/1 -> Switch/2
  signof/1 -> Bit Slice/1
  base/1 -> Switch/1, Unary Minus/1
  Switch/1 -> out/1
  Unary Minus/1 -> Switch/3

== system all_together_simu_v1/CordicAtan2/Iteration_3/X_Logic ==
  xo : Inport
  yo : Inport  Port=2
  Add2 : Sum
  Bit Shift : hdlsllib/Logic and Bit Operations/Bit Shift  mode=Shift Right Arithmetic  N=2
  zsign : Subsystem
  x : Outport
  wires:
  yo/1 -> zsign/1(signof), Bit Shift/1
  Bit Shift/1 -> zsign/2(base)
  xo/1 -> Add2/1
  Add2/1 -> x/1
  zsign/1(out) -> Add2/2  "xo"

== system all_together_simu_v1/CordicAtan2/Iteration_3/Y_Logic ==
  xo : Inport
  yo : Inport  Port=2
  Add1 : Sum  OutDataTypeStr=fixdt(1,16,15)
  Bit Shift : hdlsllib/Logic and Bit Operations/Bit Shift  mode=Shift Right Arithmetic  N=2
  n_zsign : Subsystem
  y : Outport
  wires:
  Bit Shift/1 -> n_zsign/2(base)
  n_zsign/1(out) -> Add1/2
  Add1/1 -> y/1
  xo/1 -> Bit Shift/1
  yo/1 -> n_zsign/1(signof), Add1/1

== system all_together_simu_v1/CordicAtan2/Iteration_3/n_zsign ==
  signof : Inport
  base : Inport  Port=2
  Bit Slice : hdlsllib/Logic and Bit Operations/Bit Slice  lidx=15  ridx=15
      settings: SourceProductBaseCode=SL
  Switch : Switch  Criteria=u2 > Threshold
  Unary Minus : UnaryMinus
  out : Outport
  wires:
  Bit Slice/1 -> Switch/2
  signof/1 -> Bit Slice/1
  base/1 -> Switch/1, Unary Minus/1
  Switch/1 -> out/1
  Unary Minus/1 -> Switch/3

== system all_together_simu_v1/CordicAtan2/Iteration_4/X_Logic ==
  xo : Inport
  yo : Inport  Port=2
  Add2 : Sum
  Bit Shift : hdlsllib/Logic and Bit Operations/Bit Shift  mode=Shift Right Arithmetic  N=3
  zsign : Subsystem
  x : Outport
  wires:
  yo/1 -> zsign/1(signof), Bit Shift/1
  Bit Shift/1 -> zsign/2(base)
  xo/1 -> Add2/1
  Add2/1 -> x/1
  zsign/1(out) -> Add2/2  "xo"

== system all_together_simu_v1/CordicAtan2/Iteration_4/Y_Logic ==
  xo : Inport
  yo : Inport  Port=2
  Add1 : Sum  OutDataTypeStr=fixdt(1,16,16)
  Bit Shift : hdlsllib/Logic and Bit Operations/Bit Shift  mode=Shift Right Arithmetic  N=3
  n_zsign : Subsystem
  y : Outport
  wires:
  Bit Shift/1 -> n_zsign/2(base)
  n_zsign/1(out) -> Add1/2
  Add1/1 -> y/1
  xo/1 -> Bit Shift/1
  yo/1 -> n_zsign/1(signof), Add1/1

== system all_together_simu_v1/CordicAtan2/Iteration_4/n_zsign ==
  signof : Inport
  base : Inport  Port=2
  Bit Slice : hdlsllib/Logic and Bit Operations/Bit Slice  lidx=15  ridx=15
      settings: SourceProductBaseCode=SL
  Switch : Switch  Criteria=u2 > Threshold
  Unary Minus : UnaryMinus
  out : Outport
  wires:
  Bit Slice/1 -> Switch/2
  signof/1 -> Bit Slice/1
  base/1 -> Switch/1, Unary Minus/1
  Switch/1 -> out/1
  Unary Minus/1 -> Switch/3

== system all_together_simu_v1/CordicAtan2/Iteration_5/X_Logic ==
  xo : Inport
  yo : Inport  Port=2
  Add2 : Sum
  Bit Shift : hdlsllib/Logic and Bit Operations/Bit Shift  mode=Shift Right Arithmetic  N=4
  zsign : Subsystem
  x : Outport
  wires:
  yo/1 -> zsign/1(signof), Bit Shift/1
  Bit Shift/1 -> zsign/2(base)
  xo/1 -> Add2/1
  Add2/1 -> x/1
  zsign/1(out) -> Add2/2  "xo"

== system all_together_simu_v1/CordicAtan2/Iteration_5/Y_Logic ==
  xo : Inport
  yo : Inport  Port=2
  Add1 : Sum  OutDataTypeStr=fixdt(1,16,18)
  Bit Shift : hdlsllib/Logic and Bit Operations/Bit Shift  mode=Shift Right Arithmetic  N=4
  n_zsign : Subsystem
  y : Outport
  wires:
  Bit Shift/1 -> n_zsign/2(base)
  n_zsign/1(out) -> Add1/2
  Add1/1 -> y/1
  xo/1 -> Bit Shift/1
  yo/1 -> n_zsign/1(signof), Add1/1

== system all_together_simu_v1/CordicAtan2/Iteration_5/n_zsign ==
  signof : Inport
  base : Inport  Port=2
  Bit Slice : hdlsllib/Logic and Bit Operations/Bit Slice  lidx=15  ridx=15
      settings: SourceProductBaseCode=SL
  Switch : Switch  Criteria=u2 > Threshold
  Unary Minus : UnaryMinus
  out : Outport
  wires:
  Bit Slice/1 -> Switch/2
  signof/1 -> Bit Slice/1
  base/1 -> Switch/1, Unary Minus/1
  Switch/1 -> out/1
  Unary Minus/1 -> Switch/3

== system all_together_simu_v1/CordicAtan2/Iteration_6/X_Logic ==
  xo : Inport
  yo : Inport  Port=2
  Add2 : Sum
  Bit Shift : hdlsllib/Logic and Bit Operations/Bit Shift  mode=Shift Right Arithmetic  N=5
  zsign : Subsystem
  x : Outport
  wires:
  yo/1 -> zsign/1(signof), Bit Shift/1
  Bit Shift/1 -> zsign/2(base)
  xo/1 -> Add2/1
  Add2/1 -> x/1
  zsign/1(out) -> Add2/2  "xo"

== system all_together_simu_v1/CordicAtan2/Iteration_6/Y_Logic ==
  xo : Inport
  yo : Inport  Port=2
  Add1 : Sum  OutDataTypeStr=fixdt(1,16,18)
  Bit Shift : hdlsllib/Logic and Bit Operations/Bit Shift  mode=Shift Right Arithmetic  N=5
  n_zsign : Subsystem
  y : Outport
  wires:
  Bit Shift/1 -> n_zsign/2(base)
  n_zsign/1(out) -> Add1/2
  Add1/1 -> y/1
  xo/1 -> Bit Shift/1
  yo/1 -> n_zsign/1(signof), Add1/1

== system all_together_simu_v1/CordicAtan2/Iteration_6/n_zsign ==
  signof : Inport
  base : Inport  Port=2
  Bit Slice : hdlsllib/Logic and Bit Operations/Bit Slice  lidx=15  ridx=15
      settings: SourceProductBaseCode=SL
  Switch : Switch  Criteria=u2 > Threshold
  Unary Minus : UnaryMinus
  out : Outport
  wires:
  Bit Slice/1 -> Switch/2
  signof/1 -> Bit Slice/1
  base/1 -> Switch/1, Unary Minus/1
  Switch/1 -> out/1
  Unary Minus/1 -> Switch/3

== system all_together_simu_v1/CordicAtan2/Iteration_7/X_Logic ==
  xo : Inport
  yo : Inport  Port=2
  Add2 : Sum
  Bit Shift : hdlsllib/Logic and Bit Operations/Bit Shift  mode=Shift Right Arithmetic  N=6
  zsign : Subsystem
  x : Outport
  wires:
  yo/1 -> zsign/1(signof), Bit Shift/1
  Bit Shift/1 -> zsign/2(base)
  xo/1 -> Add2/1
  Add2/1 -> x/1
  zsign/1(out) -> Add2/2  "xo"

== system all_together_simu_v1/CordicAtan2/Iteration_7/Y_Logic ==
  xo : Inport
  yo : Inport  Port=2
  Add1 : Sum  OutDataTypeStr=fixdt(1,16,19)
  Bit Shift : hdlsllib/Logic and Bit Operations/Bit Shift  mode=Shift Right Arithmetic  N=6
  n_zsign : Subsystem
  y : Outport
  wires:
  Bit Shift/1 -> n_zsign/2(base)
  n_zsign/1(out) -> Add1/2
  Add1/1 -> y/1
  xo/1 -> Bit Shift/1
  yo/1 -> n_zsign/1(signof), Add1/1

== system all_together_simu_v1/CordicAtan2/Iteration_7/n_zsign ==
  signof : Inport
  base : Inport  Port=2
  Bit Slice : hdlsllib/Logic and Bit Operations/Bit Slice  lidx=15  ridx=15
      settings: SourceProductBaseCode=SL
  Switch : Switch  Criteria=u2 > Threshold
  Unary Minus : UnaryMinus
  out : Outport
  wires:
  Bit Slice/1 -> Switch/2
  signof/1 -> Bit Slice/1
  base/1 -> Switch/1, Unary Minus/1
  Switch/1 -> out/1
  Unary Minus/1 -> Switch/3

== system all_together_simu_v1/CordicAtan2/Iteration_8/X_Logic ==
  xo : Inport
  yo : Inport  Port=2
  Add2 : Sum
  Bit Shift : hdlsllib/Logic and Bit Operations/Bit Shift  mode=Shift Right Arithmetic  N=7
  zsign : Subsystem
  x : Outport
  wires:
  yo/1 -> zsign/1(signof), Bit Shift/1
  Bit Shift/1 -> zsign/2(base)
  xo/1 -> Add2/1
  Add2/1 -> x/1
  zsign/1(out) -> Add2/2  "xo"

== system all_together_simu_v1/CordicAtan2/Iteration_8/Y_Logic ==
  xo : Inport
  yo : Inport  Port=2
  Add1 : Sum  OutDataTypeStr=fixdt(1,16,20)
  Bit Shift : hdlsllib/Logic and Bit Operations/Bit Shift  mode=Shift Right Arithmetic  N=7
  n_zsign : Subsystem
  y : Outport
  wires:
  Bit Shift/1 -> n_zsign/2(base)
  n_zsign/1(out) -> Add1/2
  Add1/1 -> y/1
  xo/1 -> Bit Shift/1
  yo/1 -> n_zsign/1(signof), Add1/1

== system all_together_simu_v1/CordicAtan2/Iteration_8/n_zsign ==
  signof : Inport
  base : Inport  Port=2
  Bit Slice : hdlsllib/Logic and Bit Operations/Bit Slice  lidx=15  ridx=15
      settings: SourceProductBaseCode=SL
  Switch : Switch  Criteria=u2 > Threshold
  Unary Minus : UnaryMinus
  out : Outport
  wires:
  Bit Slice/1 -> Switch/2
  signof/1 -> Bit Slice/1
  base/1 -> Switch/1, Unary Minus/1
  Switch/1 -> out/1
  Unary Minus/1 -> Switch/3

== system all_together_simu_v1/CordicAtan2/Iteration_9/X_Logic ==
  xo : Inport
  yo : Inport  Port=2
  Add2 : Sum
  Bit Shift : hdlsllib/Logic and Bit Operations/Bit Shift  mode=Shift Right Arithmetic  N=8
  zsign : Subsystem
  x : Outport
  wires:
  yo/1 -> zsign/1(signof), Bit Shift/1
  Bit Shift/1 -> zsign/2(base)
  xo/1 -> Add2/1
  Add2/1 -> x/1
  zsign/1(out) -> Add2/2  "xo"

== system all_together_simu_v1/CordicAtan2/Iteration_9/Y_Logic ==
  xo : Inport
  yo : Inport  Port=2
  Add1 : Sum  OutDataTypeStr=fixdt(1,16,21)
  Bit Shift : hdlsllib/Logic and Bit Operations/Bit Shift  mode=Shift Right Arithmetic  N=8
  n_zsign : Subsystem
  y : Outport
  wires:
  Bit Shift/1 -> n_zsign/2(base)
  n_zsign/1(out) -> Add1/2
  Add1/1 -> y/1
  xo/1 -> Bit Shift/1
  yo/1 -> n_zsign/1(signof), Add1/1

== system all_together_simu_v1/CordicAtan2/Iteration_9/n_zsign ==
  signof : Inport
  base : Inport  Port=2
  Bit Slice : hdlsllib/Logic and Bit Operations/Bit Slice  lidx=15  ridx=15
      settings: SourceProductBaseCode=SL
  Switch : Switch  Criteria=u2 > Threshold
  Unary Minus : UnaryMinus
  out : Outport
  wires:
  Bit Slice/1 -> Switch/2
  signof/1 -> Bit Slice/1
  base/1 -> Switch/1, Unary Minus/1
  Switch/1 -> out/1
  Unary Minus/1 -> Switch/3

== system all_together_simu_v1/CordicAtan2/Setup_Stage/n_zsign ==
  signof : Inport
  base : Inport  Port=2
  Bit Slice : hdlsllib/Logic and Bit Operations/Bit Slice  lidx=15  ridx=15
      settings: SourceProductBaseCode=SL
  Switch : Switch  Criteria=u2 > Threshold
  Unary Minus : UnaryMinus
  out : Outport
  wires:
  Bit Slice/1 -> Switch/2
  signof/1 -> Bit Slice/1
  base/1 -> Switch/1, Unary Minus/1
  Switch/1 -> out/1
  Unary Minus/1 -> Switch/3

== system all_together_simu_v1/CordicAtan2/Setup_Stage/n_zsign1 ==
  signof : Inport
  base : Inport  Port=2
  Bit Slice : hdlsllib/Logic and Bit Operations/Bit Slice  lidx=15  ridx=15
      settings: SourceProductBaseCode=SL
  Switch : Switch  Criteria=u2 > Threshold
  Unary Minus : UnaryMinus
  out : Outport
  wires:
  Bit Slice/1 -> Switch/2
  signof/1 -> Bit Slice/1
  base/1 -> Switch/1, Unary Minus/1
  Switch/1 -> out/1
  Unary Minus/1 -> Switch/3

== system all_together_simu_v1/CordicAtan2/Setup_Stage/n_zsign2 ==
  signof : Inport
  base : Inport  Port=2
  Bit Slice : hdlsllib/Logic and Bit Operations/Bit Slice  lidx=15  ridx=15
      settings: SourceProductBaseCode=SL
  Switch : Switch  Criteria=u2 > Threshold
  Unary Minus : UnaryMinus
  out : Outport
  wires:
  Bit Slice/1 -> Switch/2
  signof/1 -> Bit Slice/1
  base/1 -> Switch/1, Unary Minus/1
  Switch/1 -> out/1
  Unary Minus/1 -> Switch/3

== system all_together_simu_v1/CordicAtan2/Setup_Stage/zsign ==
  signof : Inport
  base : Inport  Port=2
  Bit Slice : hdlsllib/Logic and Bit Operations/Bit Slice  lidx=15  ridx=15
      settings: SourceProductBaseCode=SL
  Switch : Switch  Criteria=u2 > Threshold
  Unary Minus : UnaryMinus
  out : Outport
  wires:
  signof/1 -> Bit Slice/1
  Bit Slice/1 -> Switch/2
  base/1 -> Switch/3, Unary Minus/1
  Switch/1 -> out/1
  Unary Minus/1 -> Switch/1

== system all_together_simu_v1/Gradient Filter1/Horziontal Filter/ShiftReg ==
  In1 : Inport
  Enable : EnablePort
  State Control : StateControl  StateControl=Synchronous
  Tapped Delay : simulink/Discrete/Tapped Delay  vinit=0.0  samptime=-1  NumDelays=3  DelayOrder=Oldest  includeCurrent=off
  Out1 : Outport  VectorParamsAs1DForOutWhenUnconnected=off
  wires:
  In1/1 -> Tapped Delay/1
  Tapped Delay/1 -> Out1/1

== system all_together_simu_v1/Gradient Filter1/Horziontal Filter/SymmetryH ==
  In1 : Inport
  Delay18 : Delay  DelayLength=1
  Demux : Demux  Outputs=3
  Terminator : Terminator
  Terminator1 : Terminator
  Out1 : Outport  VectorParamsAs1DForOutWhenUnconnected=off
  wires:
  Demux/2 -> Delay18/1
  Demux/3 -> Terminator1/1
  Demux/1 -> Terminator/1
  Delay18/1 -> Out1/1
  In1/1 -> Demux/1

== system all_together_simu_v1/Gradient Filter1/Horziontal Filter/SymmetryV ==
  In1 : Inport
  Delay18 : Delay  DelayLength=1
  Demux : Demux  Outputs=3
  Sum3 : Sum  Inputs=|-+
  Terminator : Terminator
  Out1 : Outport  VectorParamsAs1DForOutWhenUnconnected=off
  wires:
  In1/1 -> Demux/1
  Delay18/1 -> Out1/1
  Demux/3 -> Sum3/2
  Demux/1 -> Sum3/1
  Demux/2 -> Terminator/1
  Sum3/1 -> Delay18/1

== system all_together_simu_v1/Gradient Filter1/Verticle Filter/ShiftReg ==
  In1 : Inport
  Enable : EnablePort
  State Control : StateControl  StateControl=Synchronous
  Tapped Delay : simulink/Discrete/Tapped Delay  vinit=0.0  samptime=-1  NumDelays=3  DelayOrder=Oldest  includeCurrent=off
  Out1 : Outport  VectorParamsAs1DForOutWhenUnconnected=off
  wires:
  In1/1 -> Tapped Delay/1
  Tapped Delay/1 -> Out1/1

== system all_together_simu_v1/Gradient Filter1/Verticle Filter/SymmetryH ==
  In1 : Inport
  Delay18 : Delay  DelayLength=1
  Demux : Demux  Outputs=3
  Sum3 : Sum  Inputs=|+-
  Terminator : Terminator
  Out1 : Outport  VectorParamsAs1DForOutWhenUnconnected=off
  wires:
  In1/1 -> Demux/1
  Delay18/1 -> Out1/1
  Demux/3 -> Sum3/2
  Demux/1 -> Sum3/1
  Demux/2 -> Terminator/1
  Sum3/1 -> Delay18/1

== system all_together_simu_v1/Gradient Filter1/Verticle Filter/SymmetryV ==
  In1 : Inport
  Delay18 : Delay  DelayLength=1
  Demux : Demux  Outputs=3
  Terminator : Terminator
  Terminator1 : Terminator
  Out1 : Outport  VectorParamsAs1DForOutWhenUnconnected=off
  wires:
  Demux/1 -> Terminator/1
  Demux/3 -> Terminator1/1
  Demux/2 -> Delay18/1
  In1/1 -> Demux/1
  Delay18/1 -> Out1/1

== system all_together_simu_v1/CordicAtan2/Iteration_10/X_Logic/zsign ==
  signof : Inport
  base : Inport  Port=2
  Bit Slice : hdlsllib/Logic and Bit Operations/Bit Slice  lidx=15  ridx=15
      settings: SourceProductBaseCode=SL
  Switch : Switch  Criteria=u2 > Threshold
  Unary Minus : UnaryMinus
  out : Outport
  wires:
  signof/1 -> Bit Slice/1
  Bit Slice/1 -> Switch/2
  base/1 -> Switch/3, Unary Minus/1
  Switch/1 -> out/1
  Unary Minus/1 -> Switch/1

== system all_together_simu_v1/CordicAtan2/Iteration_10/Y_Logic/n_zsign ==
  signof : Inport
  base : Inport  Port=2
  Bit Slice : hdlsllib/Logic and Bit Operations/Bit Slice  lidx=15  ridx=15
      settings: SourceProductBaseCode=SL
  Switch : Switch  Criteria=u2 > Threshold
  Unary Minus : UnaryMinus
  out : Outport
  wires:
  Bit Slice/1 -> Switch/2
  signof/1 -> Bit Slice/1
  base/1 -> Switch/1, Unary Minus/1
  Switch/1 -> out/1
  Unary Minus/1 -> Switch/3

== system all_together_simu_v1/CordicAtan2/Iteration_2/X_Logic/zsign1 ==
  signof : Inport
  base : Inport  Port=2
  Bit Slice : hdlsllib/Logic and Bit Operations/Bit Slice  lidx=15  ridx=15
      settings: SourceProductBaseCode=SL
  Switch : Switch  Criteria=u2 > Threshold
  Unary Minus : UnaryMinus
  out : Outport
  wires:
  signof/1 -> Bit Slice/1
  Bit Slice/1 -> Switch/2
  base/1 -> Switch/3, Unary Minus/1
  Switch/1 -> out/1
  Unary Minus/1 -> Switch/1

== system all_together_simu_v1/CordicAtan2/Iteration_2/Y_Logic/n_zsign ==
  signof : Inport
  base : Inport  Port=2
  Bit Slice : hdlsllib/Logic and Bit Operations/Bit Slice  lidx=15  ridx=15
      settings: SourceProductBaseCode=SL
  Switch : Switch  Criteria=u2 > Threshold
  Unary Minus : UnaryMinus
  out : Outport
  wires:
  Bit Slice/1 -> Switch/2
  signof/1 -> Bit Slice/1
  base/1 -> Switch/1, Unary Minus/1
  Switch/1 -> out/1
  Unary Minus/1 -> Switch/3

== system all_together_simu_v1/CordicAtan2/Iteration_3/X_Logic/zsign ==
  signof : Inport
  base : Inport  Port=2
  Bit Slice : hdlsllib/Logic and Bit Operations/Bit Slice  lidx=15  ridx=15
      settings: SourceProductBaseCode=SL
  Switch : Switch  Criteria=u2 > Threshold
  Unary Minus : UnaryMinus
  out : Outport
  wires:
  signof/1 -> Bit Slice/1
  Bit Slice/1 -> Switch/2
  base/1 -> Switch/3, Unary Minus/1
  Switch/1 -> out/1
  Unary Minus/1 -> Switch/1
